simulink model "Control_Block_3"  (R2021b)
settings: Solver=FixedStepAuto  StartTime=0.0  StopTime=end_time  FixedStep=dt  RelTol=1e-3
values from neighbouring files (symbols this model uses):
  Area = pi() * r0^2    [Main_PD_Control.m]    (also in Test_code.m; main.m = 1.25663706144e-05; main2.m = 1.25663706144e-05)
  Cd = 0.42    [Main_PD_Control.m]    (also in Test_code.m; main.m = 1.05; main2.m = 1.05)
  counter = time*(1/dt) +1    [Robot_system.m]    (also in main.m = 1; main2.m = 0)
  dl = l / (N - 1)    (= 0.0102040816327)    [load_parameter.m]    (also in main.m; main2.m; testcode_2d.m = 0.0204081632653)
  dt = 0.01    [Main_PD_Control.m]    (also in Test_code.m; load_parameter.m; main.m; main2.m = 0.001)
  EA = E*A    (= 13.8544236023)    [load_parameter.m]    (also in main.m; main2.m; testcode_2d.m = 10555751.3161)
  EI = E*I    (= 1.73180295029e-05)    [load_parameter.m]    (also in main.m; main2.m; testcode_2d.m = 765.291970414)
  K_d = 10    [Main_PD_Control.m]    (also in Test_code.m = 0; main.m; main2.m)
  K_p = 100    [Main_PD_Control.m]    (also in Test_code.m; main.m = 500; main2.m)
  M = zeros(2*N,2*N)    [load_parameter.m]    (also in main.m; main2.m; testcode_2d.m)
  N = length(old_posi)/2    [BoundryJudge.m]    (also in load_parameter.m = 50; main.m = 50; main2.m = 50; testcode_2d.m = 50)
  q0 = zeros(2*N,1)    [load_parameter.m]    (also in main.m; main2.m; testcode_2d.m = q)
  rho_blood = 1025    [main.m]    (also in main2.m)
  tol = EI / l^2 * 1e-3    (= 6.92721180117e-08)    [load_parameter.m]    (also in main.m; main2.m; testcode_2d.m = 0.765291970414)
settings Model: Creator=zhong  LastModifiedBy=24607
settings DebuggingCC: UnderSpecifiedDimensionMsg=error

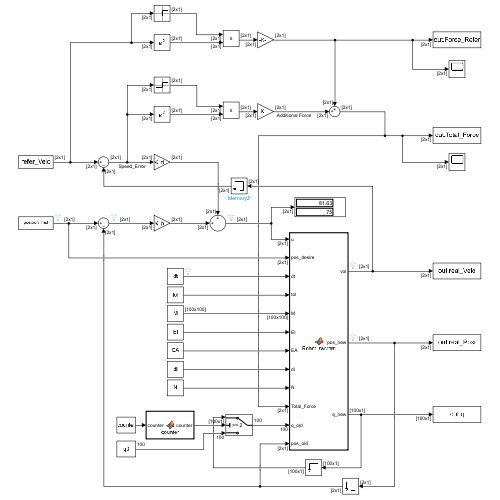
[thumbnail: Simulink's stored preview of the top-level diagram]
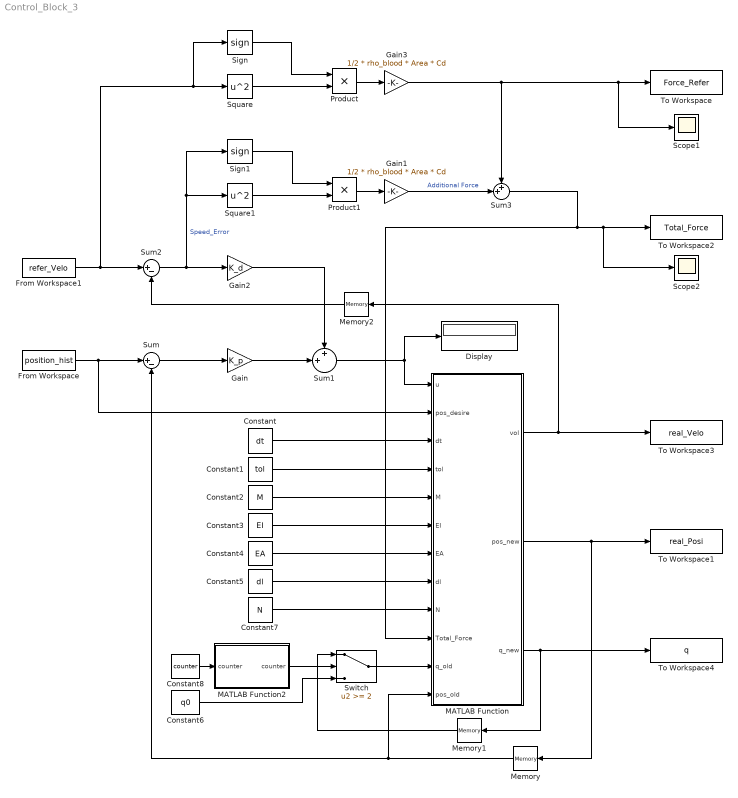
== system Control_Block_3 ==
  Constant : Constant  Value=dt
  Constant1 : Constant  Value=tol
  Constant2 : Constant  Value=M
  Constant3 : Constant  Value=EI
  Constant4 : Constant  Value=EA
  Constant5 : Constant  Value=dl
  Constant6 : Constant  Value=q0
  Constant7 : Constant  Value=N
  Constant8 : Constant  Value=counter
  Display : Display
  From Workspace : FromWorkspace  VariableName=position_hist
  From Workspace1 : FromWorkspace  VariableName=refer_Velo
  Gain : Gain  Gain=K_p
  Gain1 : Gain  Gain=1/2 * rho_blood * Area * Cd
  Gain2 : Gain  Gain=K_d
  Gain3 : Gain  Gain=1/2 * rho_blood * Area * Cd
  MATLAB Function : MATLAB Function  TreatAsAtomicUnit=on
  MATLAB Function2 : MATLAB Function  TreatAsAtomicUnit=on
  Memory : Memory
  Memory1 : Memory
  Memory2 : Memory
  Product : Product
  Product1 : Product
  Scope1 : Scope
  Scope2 : Scope
  Sign : Signum
  Sign1 : Signum
  Square : Math  Operator=square  SaturateOnIntegerOverflow=on
  Square1 : Math  Operator=square  SaturateOnIntegerOverflow=on
  Sum : Sum  Inputs=|+-
  Sum1 : Sum  Inputs=++|
  Sum2 : Sum  Inputs=|+-
  Sum3 : Sum  Inputs=++|
  Switch : Switch  Threshold=2
  To Workspace : ToWorkspace  VariableName=Force_Refer  SaveFormat=Structure With Time  SampleTime=-1
  To Workspace1 : ToWorkspace  VariableName=real_Posi  SaveFormat=Timeseries  SampleTime=-1
  To Workspace2 : ToWorkspace  VariableName=Total_Force  SaveFormat=Timeseries  SampleTime=-1
  To Workspace3 : ToWorkspace  VariableName=real_Velo  SaveFormat=Timeseries  SampleTime=-1
  To Workspace4 : ToWorkspace  VariableName=q  SaveFormat=Timeseries  SampleTime=-1
  wires:
  From Workspace/1 -> MATLAB Function/2(pos_desire), Sum/1
  Sum/1 -> Gain/1
  Gain/1 -> Sum1/2
  Sum2/1 -> Sign1/1, Square1/1, Gain2/1  "Speed_Error"
  Gain2/1 -> Sum1/1
  Sum1/1 -> Display/1, MATLAB Function/1(u)
  From Workspace1/1 -> Sum2/1, Sign/1, Square/1
  Sum3/1 -> MATLAB Function/10(Total_Force), Scope2/1, To Workspace2/1
  Constant/1 -> MATLAB Function/3(dt)
  MATLAB Function/2(pos_new) -> To Workspace1/1, Memory/1
  MATLAB Function/1(vol) -> Memory2/1, To Workspace3/1
  Gain3/1 -> Sum3/1, Scope1/1, To Workspace/1
  Gain1/1 -> Sum3/2  "Additional Force"
  Square/1 -> Product/2
  Sign/1 -> Product/1
  Product/1 -> Gain3/1
  Sign1/1 -> Product1/1
  Square1/1 -> Product1/2
  Product1/1 -> Gain1/1
  Constant8/1 -> MATLAB Function2/1("counter ")
  Constant3/1 -> MATLAB Function/6(EI)
  Constant4/1 -> MATLAB Function/7(EA)
  Constant5/1 -> MATLAB Function/8(dl)
  Constant7/1 -> MATLAB Function/9(N)
  Constant2/1 -> MATLAB Function/5(M)
  Constant1/1 -> MATLAB Function/4(tol)
  MATLAB Function2/1(counter) -> Switch/2
  Constant6/1 -> Switch/3
  MATLAB Function/3(q_new) -> To Workspace4/1, Memory1/1
  Switch/1 -> MATLAB Function/11(q_old)
  Memory/1 -> Sum/2, MATLAB Function/12(pos_old)
  Memory1/1 -> Switch/1
  Memory2/1 -> Sum2/2

== matlab function Control_Block_3/MATLAB Function ==
  data: vol output; u input; pos_desire input; dt input; tol input; M input; EI input; EA input; dl input; N input; Total_Force input; q_old input; pos_old input; pos_new output; q_new output
function [vol,pos_new,q_new]= Robot_system(u,pos_desire,dt,tol,M,EI,EA,dl,N,Total_Force,q_old,pos_old)

Ex_force = zeros(2*N,1);

    q = q_old; % Guess
    vel = (q - q_old) / dt;
    q(1:2) = (pos_desire + u)';
    
    err = 10 * tol;
     % Newton Raphson
    while err > tol

    % Inertia 
    f = M/ dt * ((q - q_old) / dt - vel);
    J = M/ dt^2;

    % Elastic forces 
    % Linear Spring 
    for k = 1: N-1
        xk = q(2*k-1);
        yk = q(2*k);
        xkp1 = q(2*k+1);
        ykp1 = q(2*k+2); 
        dF = gradEs(xk, yk, xkp1, ykp1, dl, EA);
        dJ = hessEs(xk, yk, xkp1, ykp1, dl, EA);
        f(2*k-1:2*k+2) = f(2*k-1:2*k+2) + dF;
        J(2*k-1:2*k+2, 2*k-1:2*k+2) = ...
        J(2*k-1:2*k+2, 2*k-1:2*k+2) + dJ;
    end

    % Bending spring 
    for k = 2:N-1
        xkm1 = q(2*k-3);
        ykm1 = q(2*k-2);
        xk = q(2*k-1);
        yk = q(2*k);
        xkp1 = q(2*k+1);
        ykp1 = q(2*k+2);
        curvature0 = 0;
        dF = gradEb(xkm1, ykm1, xk, yk, xkp1, ykp1, curvature0, dl, EI);
        dJ = hessEb(xkm1, ykm1, xk, yk, xkp1, ykp1, curvature0, dl, EI);
        f(2*k-3:2*k+2) = f(2*k-3:2*k+2) + dF;
        J(2*k-3:2*k+2, 2*k-3:2*k+2) = ...
            J(2*k-3:2*k+2, 2*k-3:2*k+2) + dJ;
    end
    % External force 
    Ex_force(1) = Total_Force(1,:);
    Ex_force(2) = Total_Force(2,:);

    f = f + Ex_force;

    q(1:(2*N)) = q(1:(2*N)) - J(1:(2*N),1:(2*N)) \ f(1:(2*N));
    err = sum(abs(f(1:(2*N))));
    end

    pos_new = q(1:2,:);
    q_new = q;
    vol = (pos_new - pos_old)/dt;

== matlab function Control_Block_3/MATLAB Function2 ==
  data: counter input; counter output
function counter = counter(counter)

counter = counter + 1;
